simulink model "Simulink_10"  (Simulink 10.0)
settings: Solver=ode45  StartTime=0.0  StopTime=200.0  RelTol=1e-6  AbsTol=1e-6  EnableMultiTasking=on
StopFcn:
  | % plot from t=50 to the end
  | for i=1:length(tout)
  |   if(tout(i)) >= 50
  |     break
  |   end
  | end
  | plot(yout(i:end,5),yout(i:end,8), 'r')
  | axis square
libraries: simulink x1
settings Model: Creator=stephen  LastModifiedBy=unknown
settings SolverCC: AutoScaleAbsTol=off  ZeroCrossControl=DisableAll  ZeroCrossAlgorithm=Non-adaptive
settings DataIOCC: SignalLoggingSaveFormat=ModelDataLogs  SignalLoggingName=sigsOut
settings OptimizationCC: ExpressionDepthLimit=2147483647  InitFltsAndDblsToZero=on
settings DebuggingCC: SaveWithParameterizedLinksMsg=none  SignalResolutionControl=TryResolveAllWithWarning  MultiTaskDSMMsg=warning  MultiTaskCondExecSysMsg=none  FcnCallInpInsideContextMsg=warning  StateNameClashWarn=warning
settings HardwareCC: TargetUnknown=on
settings SFSimCC: SimUseLocalCustomCode=on  CustomCodeUndefinedFunction=FilterOut
settings RTWCC: RTWUseLocalCustomCode=on
settings GRTTargetCC: ModelReferenceCompliant=off  CompOptLevelCompliant=off  MatFileLogging=off

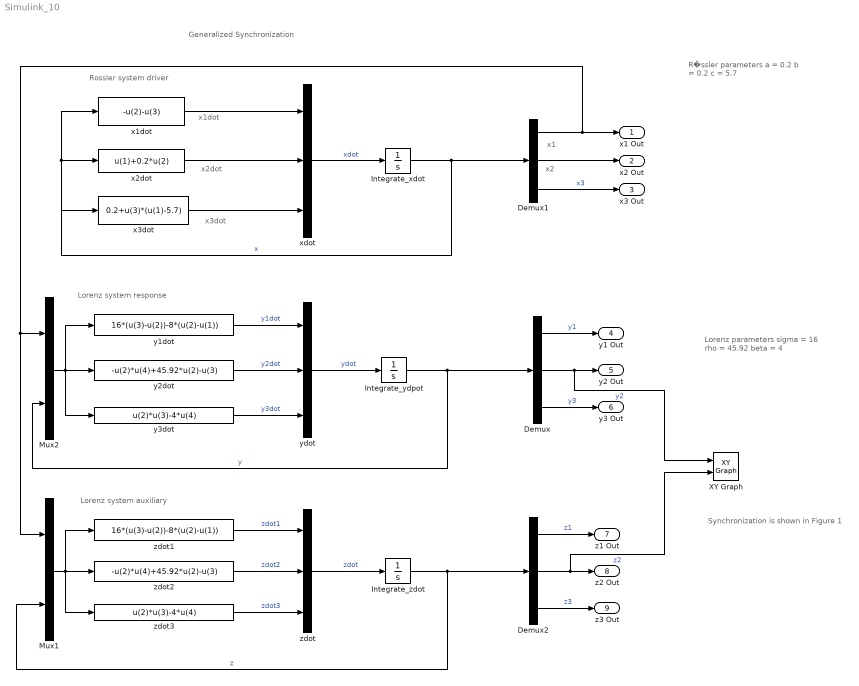
== system Simulink_10 ==
  note: Generalized Synchronization
  note: R�ssler parameters
      | a = 0.2
      | b = 0.2
      | c = 5.7
  note: x1dot
  note: x2dot
  note: x3dot
  note: x2
  note: x1
  note: Lorenz system response
  note: Lorenz system auxiliary
  note: Lorenz parameters
      | sigma = 16
      | rho = 45.92
      | beta = 4
  note: Rossler system driver
  note: Synchronization is shown in Figure 1
  Demux : Demux  Outputs=3
  Demux1 : Demux  Outputs=3
  Demux2 : Demux  Outputs=3
  Integrate_xdot : Integrator  InitialCondition=[2 -10 44]  UpperSaturationLimit=50  LowerSaturationLimit=0  ContinuousStateAttributes='x'
  Integrate_ydpot : Integrator  InitialCondition=[30 10 20]  UpperSaturationLimit=50  LowerSaturationLimit=0  ContinuousStateAttributes='y'
  Integrate_zdot : Integrator  InitialCondition=[31 11 22 ]  UpperSaturationLimit=50  LowerSaturationLimit=0
  Mux1 : Mux  Inputs=[1 3]
  Mux2 : Mux  Inputs=[1 3]
  XY Graph : simulink/Sinks/XY Graph  SystemSampleTime=-1  xmin=-50  xmax=50  ymin=-50  ymax=50  st=-1
  x1dot : Fcn  Description=sdhdkbkdf  Expr=-u(2)-u(3)
  x2dot : Fcn  Expr=u(1)+0.2*u(2)
  x3dot : Fcn  Expr=0.2+u(3)*(u(1)-5.7)
  xdot : Mux  Inputs=3
  y1dot : Fcn  Description=sdhdkbkdf  Expr=16*(u(3)-u(2))-8*(u(2)-u(1))
  y2dot : Fcn  Expr=-u(2)*u(4)+45.92*u(2)-u(3)
  y3dot : Fcn  Expr=u(2)*u(3)-4*u(4)
  ydot : Mux  Inputs=3
  zdot : Mux  Inputs=3
  zdot1 : Fcn  Description=sdhdkbkdf  Expr=16*(u(3)-u(2))-8*(u(2)-u(1))
  zdot2 : Fcn  Expr=-u(2)*u(4)+45.92*u(2)-u(3)
  zdot3 : Fcn  Expr=u(2)*u(3)-4*u(4)
  x1 Out : Outport
  x2 Out : Outport  Port=2
  x3 Out : Outport  Port=3
  y1 Out : Outport  Port=4
  y2 Out : Outport  Port=5
  y3 Out : Outport  Port=6
  z1 Out : Outport  Port=7
  z2 Out : Outport  Port=8
  z3 Out : Outport  Port=9
  wires:
  ydot/1 -> Integrate_ydpot/1  "ydot"
  x1dot/1 -> xdot/1
  x2dot/1 -> xdot/2
  x3dot/1 -> xdot/3
  xdot/1 -> Integrate_xdot/1  "xdot"
  Integrate_xdot/1 -> x2dot/1, x1dot/1, x3dot/1, Demux1/1  "x"
  y3dot/1 -> ydot/3  "y3dot"
  y2dot/1 -> ydot/2  "y2dot"
  y1dot/1 -> ydot/1  "y1dot"
  zdot/1 -> Integrate_zdot/1  "zdot"
  Demux1/2 -> x2 Out/1
  Demux1/3 -> x3 Out/1  "x3"
  Demux1/1 -> x1 Out/1, Mux2/1, Mux1/1
  Demux2/3 -> z3 Out/1  "z3"
  Demux/3 -> y3 Out/1  "y3"
  Demux/1 -> y1 Out/1  "y1"
  Demux2/1 -> z1 Out/1  "z1"
  Demux2/2 -> XY Graph/2, z2 Out/1  "z2"
  Demux/2 -> XY Graph/1, y2 Out/1  "y2"
  Mux2/1 -> y2dot/1, y1dot/1, y3dot/1
  Integrate_ydpot/1 -> Demux/1, Mux2/2  "y"
  Integrate_zdot/1 -> Demux2/1, Mux1/2  "z"
  zdot1/1 -> zdot/1  "zdot1"
  zdot2/1 -> zdot/2  "zdot2"
  zdot3/1 -> zdot/3  "zdot3"
  Mux1/1 -> zdot2/1, zdot1/1, zdot3/1
